simulink model "LQG_inner_loop"  (R2024b)
settings: Solver=VariableStepAuto  StartTime=0.0  StopTime=misc.T  RelTol=1e-3
undefined symbols (not defined in the file): act, body, ctrl, guid, height, ic, nav
libraries: simulink x2, simulink_extras x1
settings Model: Creator=Eliot Nychka  LastModifiedBy=devin
settings DebuggingCC: AlgebraicLoopMsg=none

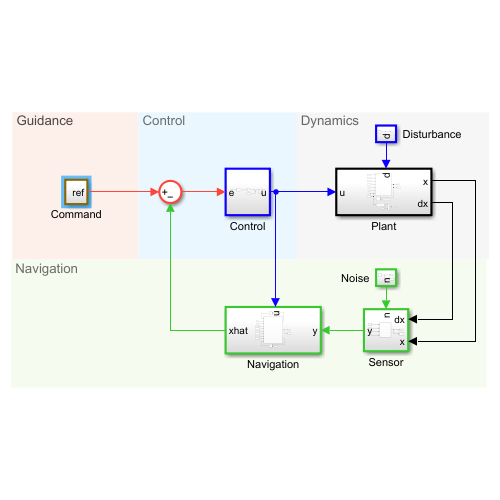
[thumbnail: Simulink's stored preview of the top-level diagram]
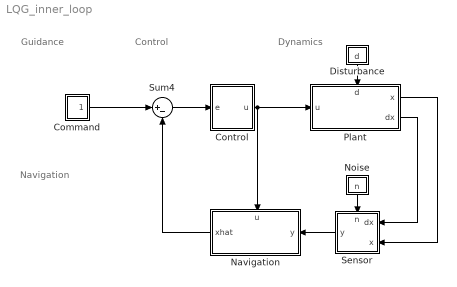
== system LQG_inner_loop ==
  note: Navigation
  note: Dynamics
  note: Guidance
  note: Control
  Command : Subsystem
  Control : Subsystem
  Disturbance : Subsystem
  Navigation : Subsystem
      settings: PortSchema="{\"entries\":[{\"content\":{\"sides\":[{\"content\":{\"connectorIds\":[\"In1\"]},\"type\":\"ConnectorPlacement.EquallySpacedRectSide\",\"uuid\":\"ed9a3bfc-e7a2-4410-871f-111b32929a82\"},{\"content\":{\"connectorIds\":[\"Out1\"],\"side\":\"RIGHT\"},\"type\":\"ConnectorPlacement.EquallySpacedRectSide\",\"uuid\":\"9caadf78-b71d-47f7-a4d6-15bfba055fff\"},{\"content\":{\"connectorIds\":[\"In2\"],\"side\":\"TOP\"},\"type\":\"ConnectorPlacement.EquallySpacedRectSide\",\"uuid\":\"b88ce8b4-fb25-4be5-b583-e8b5fea62f77\"}]},\"type\":\"ConnectorPlacement.EquallySpacedConnector\",\"uuid\":\"b8a90069-3825-4fdb-922d-4002bd1daead\"}],\"packageUris\":[\"http://schema.mathworks.com/mf0/Connector/R2020b\"],\"version\":\"1.0\"}"
  Noise : Subsystem
  Plant : Subsystem
      settings: PortSchema="{\"entries\":[{\"content\":{\"sides\":[{\"content\":{\"connectorIds\":[\"In1\"]},\"type\":\"ConnectorPlacement.EquallySpacedRectSide\",\"uuid\":\"53915b1a-b285-44c5-8350-0c9f1bc1b8aa\"},{\"content\":{\"connectorIds\":[\"Out1\",\"Out2\"],\"side\":\"RIGHT\"},\"type\":\"ConnectorPlacement.EquallySpacedRectSide\",\"uuid\":\"1ce863af-0af9-488c-b338-1118d88ebce9\"},{\"content\":{\"connectorIds\":[\"In2\"],\"side\":\"TOP\"},\"type\":\"ConnectorPlacement.EquallySpacedRectSide\",\"uuid\":\"1cd27b0c-b3c0-43f5-9d46-63ebc1724ecf\"}]},\"type\":\"ConnectorPlacement.EquallySpacedConnector\",\"uuid\":\"51ba1034-53e0-4b22-a802-13a5cc6d5773\"}],\"packageUris\":[\"http://schema.mathworks.com/mf0/Connector/R2020b\"],\"version\":\"1.0\"}"
  Sensor : Subsystem
      settings: PortSchema="{\"entries\":[{\"content\":{\"sides\":[{\"content\":{\"connectorIds\":[\"In1\",\"In2\"]},\"type\":\"ConnectorPlacement.EquallySpacedRectSide\",\"uuid\":\"c10a2f4f-01ed-46cf-9353-9999ca068f80\"},{\"content\":{\"connectorIds\":[\"Out1\"],\"side\":\"RIGHT\"},\"type\":\"ConnectorPlacement.EquallySpacedRectSide\",\"uuid\":\"1bf68d2b-7a9c-4702-b99e-db3ed675bf63\"},{\"content\":{\"connectorIds\":[\"In3\"],\"side\":\"TOP\"},\"type\":\"ConnectorPlacement.EquallySpacedRectSide\",\"uuid\":\"a38c0bfa-50ca-443b-8f9e-c3be6d337dc6\"},{\"content\":{\"side\":\"BOTTOM\"},\"type\":\"ConnectorPlacement.EquallySpacedRectSide\",\"uuid\":\"e991ef87-5088-4ee0-859c-08a45d39029e\"}]},\"type\":\"ConnectorPlacement.EquallySpacedConnector\",\"uuid\":\"d1858c6f-fee5-45e0-983d-3d9154617473\"}],\"packageUris\":[\"http://schema.mathworks.com/mf0/Connector/R2020b\"],\"version\":\"1.0\"}"
  Sum4 : Sum  Inputs=|+-
  wires:
  Plant/1(x) -> Sensor/2(x)
  Control/1(u) -> Navigation/2(u), Plant/1(u)
  Sum4/1 -> Control/1(e)
  Command/1(ref) -> Sum4/1
  Plant/2(dx) -> Sensor/1(dx)
  Noise/1(n) -> Sensor/3(n)
  Disturbance/1(d) -> Plant/2(d)
  Sensor/1(y) -> Navigation/1(y)
  Navigation/1(xhat) -> Sum4/2

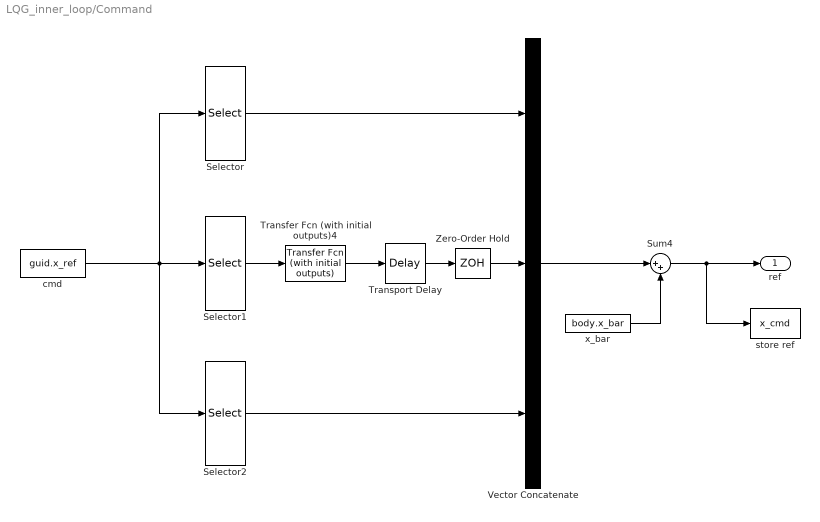
== system LQG_inner_loop/Command ==
  Selector : Selector  InputPortWidth=13  IndexOptions=Index vector (dialog)  Indices=[1 2 3]  OutputSizes=1
  Selector1 : Selector  InputPortWidth=13  IndexOptions=Index vector (dialog)  Indices=4  OutputSizes=1
  Selector2 : Selector  InputPortWidth=13  IndexOptions=Index vector (dialog)  Indices=[5:13]  OutputSizes=1
  Sum4 : Sum  Inputs=|++
  Transfer Fcn (with initial outputs)4 : simulink_extras/Additional Linear/Transfer Fcn (with initial outputs)  N=[1]  D="[4  1]"  Y0=0  U0=0
  Transport Delay : TransportDelay  DelayTime=5
  Vector Concatenate : Concatenate  NumInputs=3  Mode=Multidimensional array
  Zero-Order Hold : ZeroOrderHold  SampleTime=nav.T
  cmd : Constant  Value=guid.x_ref  SampleTime=guid.T
  store ref : ToWorkspace  VariableName=x_cmd  SaveFormat=Timeseries  SampleTime=guid.T
  x_bar : Constant  Value=body.x_bar  SampleTime=guid.T
  ref : Outport  SampleTime=guid.T
  wires:
  Selector1/1 -> Transfer Fcn (with initial outputs)4/1
  Sum4/1 -> store ref/1, ref/1
  Selector/1 -> Vector Concatenate/1
  Transfer Fcn (with initial outputs)4/1 -> Transport Delay/1
  cmd/1 -> Selector1/1, Selector2/1, Selector/1
  Selector2/1 -> Vector Concatenate/3
  Vector Concatenate/1 -> Sum4/1
  x_bar/1 -> Sum4/2
  Transport Delay/1 -> Zero-Order Hold/1
  Zero-Order Hold/1 -> Vector Concatenate/2

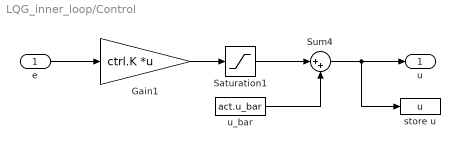
== system LQG_inner_loop/Control ==
  e : Inport  SampleTime=ctrl.T
  Gain1 : Gain  Gain=ctrl.K  Multiplication=Matrix(K*u) (u vector)
  Saturation1 : Saturate  UpperLimit=act.upper  LowerLimit=act.lower
  Sum4 : Sum  Inputs=|++
  store u : ToWorkspace  VariableName=u  SaveFormat=Timeseries  SampleTime=-1
  u_bar : Constant  Value=act.u_bar  SampleTime=ctrl.T
  u : Outport
  wires:
  Gain1/1 -> Saturation1/1
  e/1 -> Gain1/1
  Sum4/1 -> u/1, store u/1
  Saturation1/1 -> Sum4/1
  u_bar/1 -> Sum4/2

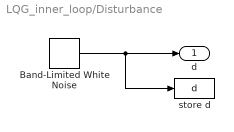
== system LQG_inner_loop/Disturbance ==
  Band-Limited White Noise : simulink/Sources/Band-Limited White Noise  Cov=ones(height(nav.Q),1)*10e-10  Ts=ctrl.T  seed=[23341]
  store d : ToWorkspace  VariableName=d  SaveFormat=Timeseries  SampleTime=-1
  d : Outport
  wires:
  Band-Limited White Noise/1 -> store d/1, d/1

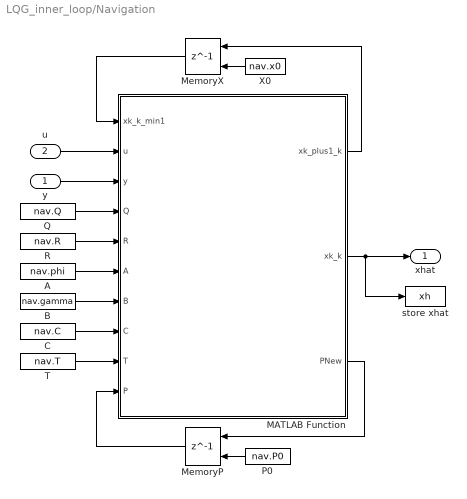
== system LQG_inner_loop/Navigation ==
  y : Inport
  u : Inport  Port=2  SampleTime=nav.T
  A : Constant  Value=nav.phi  VectorParams1D=off  OutDataTypeStr=Inherit: Inherit via back propagation  SampleTime=nav.T
  B : Constant  Value=nav.gamma  VectorParams1D=off  OutDataTypeStr=Inherit: Inherit via back propagation  SampleTime=nav.T
  C : Constant  Value=nav.C  VectorParams1D=off  OutDataTypeStr=Inherit: Inherit via back propagation  SampleTime=nav.T
  MATLAB Function : MATLAB Function  TreatAsAtomicUnit=on
  MemoryP : Delay  DelayLength=1  InitialConditionSource=Input port  SampleTime=nav.T
      settings: InputPortMap=u0,p4
  MemoryX : Delay  DelayLength=1  InitialConditionSource=Input port  SampleTime=nav.T
      settings: InputPortMap=u0,p4
  P0 : Constant  Value=nav.P0  OutDataTypeStr=Inherit: Inherit via back propagation  SampleTime=nav.T
  Q : Constant  Value=nav.Q  VectorParams1D=off  OutDataTypeStr=Inherit: Inherit via back propagation  SampleTime=nav.T
  R : Constant  Value=nav.R  VectorParams1D=off  OutDataTypeStr=Inherit: Inherit via back propagation  SampleTime=nav.T
  T : Constant  Value=nav.T  VectorParams1D=off  OutDataTypeStr=Inherit: Inherit via back propagation  SampleTime=nav.T
  X0 : Constant  Value=nav.x0  VectorParams1D=off  OutDataTypeStr=Inherit: Inherit via back propagation  SampleTime=nav.T
  store xhat : ToWorkspace  VariableName=xh  SaveFormat=Timeseries  SampleTime=-1
  xhat : Outport  VectorParamsAs1DForOutWhenUnconnected=off
  wires:
  MemoryP/1 -> MATLAB Function/10(P)
  Q/1 -> MATLAB Function/4(Q)
  P0/1 -> MemoryP/2
  MATLAB Function/3(PNew) -> MemoryP/1
  R/1 -> MATLAB Function/5(R)
  X0/1 -> MemoryX/2
  MemoryX/1 -> MATLAB Function/1(xk_k_min1)
  MATLAB Function/1(xk_plus1_k) -> MemoryX/1
  MATLAB Function/2(xk_k) -> xhat/1, store xhat/1
  A/1 -> MATLAB Function/6(A)
  B/1 -> MATLAB Function/7(B)
  C/1 -> MATLAB Function/8(C)
  T/1 -> MATLAB Function/9(T)
  u/1 -> MATLAB Function/2(u)
  y/1 -> MATLAB Function/3(y)

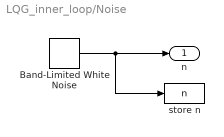
== system LQG_inner_loop/Noise ==
  Band-Limited White Noise : simulink/Sources/Band-Limited White Noise  Cov=ones(height(nav.R),1)*10e-9  Ts=nav.T  seed=[23341]
  store n : ToWorkspace  VariableName=n  SaveFormat=Timeseries  SampleTime=-1
  n : Outport
  wires:
  Band-Limited White Noise/1 -> store n/1, n/1

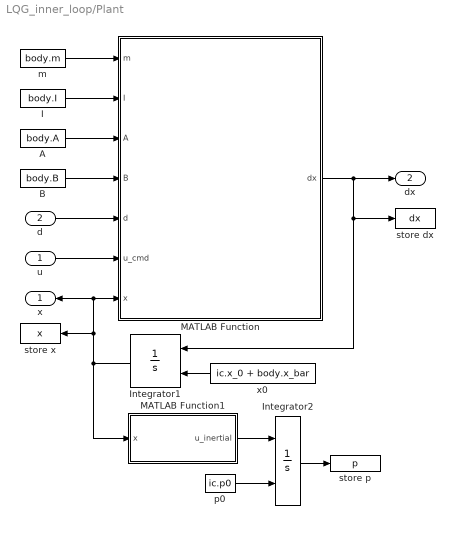
== system LQG_inner_loop/Plant ==
  u : Inport
  d : Inport  Port=2
  "A " : Constant  Value=body.A
  B : Constant  Value=body.B
  I : Constant  Value=body.I
  Integrator1 : Integrator  InitialConditionSource=external
  Integrator2 : Integrator  InitialConditionSource=external
  MATLAB Function : MATLAB Function  TreatAsAtomicUnit=on
  MATLAB Function1 : MATLAB Function  TreatAsAtomicUnit=on
  m : Constant  Value=body.m
  p0 : Constant  Value=ic.p0
  store dx : ToWorkspace  VariableName=dx  SaveFormat=Timeseries  SampleTime=-1
  store p : ToWorkspace  VariableName=p  SaveFormat=Timeseries  SampleTime=-1
  store x : ToWorkspace  VariableName=x  SaveFormat=Timeseries  SampleTime=-1
  x0 : Constant  Value=ic.x_0 + body.x_bar
  x : Outport
  dx : Outport  Port=2
  wires:
  m/1 -> MATLAB Function/1(m)
  I/1 -> MATLAB Function/2(I)
  u/1 -> MATLAB Function/6(u_cmd)
  "A "/1 -> MATLAB Function/3(A)
  B/1 -> MATLAB Function/4(B)
  x0/1 -> Integrator1/2
  d/1 -> MATLAB Function/5(d)
  MATLAB Function/1(dx) -> Integrator1/1, store dx/1, dx/1
  MATLAB Function1/1(u_inertial) -> Integrator2/1
  Integrator2/1 -> store p/1
  Integrator1/1 -> MATLAB Function1/1(x), x/1, MATLAB Function/7(x), store x/1
  p0/1 -> Integrator2/2

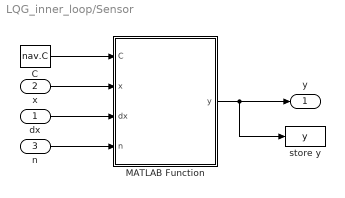
== system LQG_inner_loop/Sensor ==
  dx : Inport  SampleTime=nav.T
  x : Inport  Port=2  SampleTime=nav.T
  n : Inport  Port=3
  C : Constant  Value=nav.C  SampleTime=nav.T
  MATLAB Function : MATLAB Function  TreatAsAtomicUnit=on
  store y : ToWorkspace  VariableName=y  SaveFormat=Timeseries  SampleTime=-1
  y : Outport
  wires:
  x/1 -> MATLAB Function/2(x)
  dx/1 -> MATLAB Function/3(dx)
  n/1 -> MATLAB Function/4(n)
  MATLAB Function/1(y) -> y/1, store y/1
  C/1 -> MATLAB Function/1(C)

== matlab function LQG_inner_loop/Plant/MATLAB Function ==
  data: m input; I input; A input; B input; d input; u_cmd input; x input; dx output
function dx =  NonlinearDynamics(m, I, A, B, d, u_cmd, x)
% body properties: I, m
% actuator dynamics: A, B
% input: x, u, d 
% output: dx

% rotation matrix from inertial to body frame
T1 = [1 0 0; 0 cos(x(1)) sin(x(1)); 0 -sin(x(1)) cos(x(1))];
T2 = [cos(x(2)) 0 -sin(x(2)); 0 1 0; sin(x(2)) 0 cos(x(2))];
T3 = [cos(x(3)) sin(x(3)) 0; -sin(x(3)) cos(x(3)) 0; 0 0 1];

% dx from coupled dynamics
dx = zeros(length(x),1);
dx(1:3) = x(7:9);
dx(4:6) = cross(x(4:6),x(7:9))/m + T1*T2*T3*[-9.81; 0; 0];
dx(7:9) = I\cross([x(7:9)],I*[x(7:9)]);

% dx from actuators, disturbance
dx = dx + A(:,10:end)*x(10:end) + B*u_cmd;
dx = dx + d;

== matlab function LQG_inner_loop/Sensor/MATLAB Function ==
  data: C input; x input; y output; dx input; n input
function y = Pixhawk(C, x, dx, n)

% will be able to get x
% integrating dx (imu data) can give some states,
% gps / pitot tubes could give some states directly, etc.
% may or may not be able to measure thrusts

y = C*x + n;

== matlab function LQG_inner_loop/Navigation/MATLAB Function ==
  data: xk_k_min1 input; xk_plus1_k output; u input; y input; Q input; R input; A input; B input; C input; T input; P input; xk_k output; PNew output
function [xk_plus1_k, xk_k, PNew] = KalmanFilter(xk_k_min1, u, y, Q, R, A, B, C, T, P)
% Parameters
%   T        - Sampling Time
%   y, u     - Measurements, Control Signal
%   A, B, C  - System Matrices
%   Q, R     - Noise Covariance Matrices
%   L        - Kalman gain to get x[k+1|k] from x[k|k-1] and y[k]
%   M        - Kalman gain to get x[k|k] from x[k|k-1] and y[k]
%   Z        - State estimation covariance of x[k|k]
%   PNew     - P[k+1], state estimation error covariance for next time step
%   x[k+1|k] - from x[k|k-1] and y[k], feedback to kalman filter
%   x[k|k]   - from x[k|k-1] and y[k], output to controller

% Kalman Gains
L = A*P*C.' / (C*P*C.'+R);      
M =   P*C.' / (C*P*C.'+R);

% Covariances
Abar = eye(size(A,1),'like', A) - M*C;
Z = Abar*P*Abar.' + M*R*M.';
PNew = A*Z*A.' + Q;

% State Estimates
g = zeros(13,1); g(4) = -9.81*T;
xk_plus1_k = A*xk_k_min1 + g + B*(u) + L*(y - C*xk_k_min1);
xk_k       =   xk_k_min1 +             M*(y - C*xk_k_min1);
end

== matlab function LQG_inner_loop/Plant/MATLAB Function1 ==
  data: x input; u_inertial output
function u_inertial = BodyToInertial(x)

% body frame position
u_body = x(4:6,:); % body frame position

% inertial frame position
T1 = [1 0 0; 0 cos(x(1)) sin(x(1)); 0 -sin(x(1)) cos(x(1))];
T2 = [cos(x(2)) 0 -sin(x(2)); 0 1 0; sin(x(2)) 0 cos(x(2))];
T3 = [cos(x(3)) sin(x(3)) 0; -sin(x(3)) cos(x(3)) 0; 0 0 1];
u_inertial = (T1*T2*T3)'*u_body;

end
